simulink model "lab2_5"  (Simulink 7.9)
settings: Solver=ode45  StartTime=3  StopTime=4  RelTol=1e-3
libraries: simulink x1
settings Model: Creator=Aquirel  LastModifiedBy=Aquirel

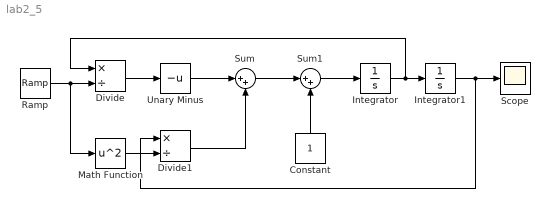
== system lab2_5 ==
  Constant : Constant
  Divide : Product  Inputs=*/
  Divide1 : Product  Inputs=*/
  Integrator : Integrator  InitialCondition=3
  Integrator1 : Integrator  InitialCondition=6
  Math Function : Math  Operator=square  SaturateOnIntegerOverflow=on
  Ramp : simulink/Sources/Ramp  slope=1  start=0  X0=0
  Scope : Scope
      settings: YMin=0  YMax=900
  Sum : Sum  Inputs=|++
  Sum1 : Sum  Inputs=|++
  Unary Minus : UnaryMinus
  wires:
  Ramp/1 -> Divide/2, Math Function/1
  Divide/1 -> Unary Minus/1
  Unary Minus/1 -> Sum/1
  Divide1/1 -> Sum/2
  Math Function/1 -> Divide1/2
  Constant/1 -> Sum1/2
  Sum/1 -> Sum1/1
  Sum1/1 -> Integrator/1
  Integrator/1 -> Divide/1, Integrator1/1
  Integrator1/1 -> Divide1/1, Scope/1
